simulink model "MCVT_v6_shell"  (R2021b)
settings: Solver=FixedStepAuto  StartTime=0.0  StopTime=1000000  FixedStep=1/fz  RelTol=1e-3
undefined symbols (not defined in the file or in its folder): fz_3
libraries: lib_subframe x71, slrealtimeutilitieslib x30, lib_header x15, slrealtimeiplib x15
(part 2 of 2)

== matlab function MCVT_v6_shell/Sys3_Power/Sys3_FDDs/3003003 ==
  settings: updateMethod=DISCRETE  sampleTime=1/fz_3
  data: fddmeas output
function fddmeas = FDD_model()

    fddmeas = rand(1,1);
    
end

== matlab function MCVT_v6_shell/Sys2_Structure/Sys2_Sensors/2002 ==
  settings: updateMethod=DISCRETE  sampleTime=1/fz_2
  data: meas output; fdd1 output; fdd2 output; fdd3 output
function [meas, fdd1, fdd2, fdd3] = Sensor_Model()
    
    meas = rand();
    fdd1 = randi([0 1]);
    fdd2 = rand();
    fdd3 = randi([0 1]);
    
end

== matlab function MCVT_v6_shell/Sys2_Structure/Sys2_Sensors/2005 ==
  settings: updateMethod=DISCRETE  sampleTime=1/fz_2
  data: meas output; fdd1 output; fdd2 output; fdd3 output
function [meas, fdd1, fdd2, fdd3] = Sensor_Model()
    
    meas = rand();
    fdd1 = randi([0 1]);
    fdd2 = rand();
    fdd3 = randi([0 1]);
    
end

== matlab function MCVT_v6_shell/Sys3_Power/Sys3_FDDs/3003004 ==
  settings: updateMethod=DISCRETE  sampleTime=1/fz_3
  data: fddmeas output
function fddmeas = FDD_model()

    fddmeas = rand(1,1);
    
end

== matlab function MCVT_v6_shell/Sys5_ECLSS/Sys5_FDDs/5002002 ==
  settings: updateMethod=DISCRETE  sampleTime=1/fz_5
  data: fddmeas output
function fddmeas = FDD_model()

    fddmeas = rand(1,1);
    
end

== matlab function MCVT_v6_shell/Sys3_Power/Sys3_Sensors/3004 ==
  settings: updateMethod=DISCRETE  sampleTime=1/fz_3
  data: meas output; fdd1 output; fdd2 output; fdd3 output
function [meas, fdd1, fdd2, fdd3] = Sensor_Model()
    
    meas = rand();
    fdd1 = randi([0 1]);
    fdd2 = rand();
    fdd3 = randi([0 1]);
    
end

== matlab function MCVT_v6_shell/Sys3_Power/Sys3_Sensors/3005 ==
  settings: updateMethod=DISCRETE  sampleTime=1/fz_3
  data: meas output; fdd1 output; fdd2 output; fdd3 output
function [meas, fdd1, fdd2, fdd3] = Sensor_Model()
    
    meas = rand();
    fdd1 = randi([0 1]);
    fdd2 = rand();
    fdd3 = randi([0 1]);
    
end

== matlab function MCVT_v6_shell/Sys3_Power/Sys3_Sensors/3006 ==
  settings: updateMethod=DISCRETE  sampleTime=1/fz_3
  data: meas output; fdd1 output; fdd2 output; fdd3 output
function [meas, fdd1, fdd2, fdd3] = Sensor_Model()
    
    meas = rand();
    fdd1 = randi([0 1]);
    fdd2 = rand();
    fdd3 = randi([0 1]);
    
end

== matlab function MCVT_v6_shell/Sys2_Structure/Sys2_Sensors/2006 ==
  settings: updateMethod=DISCRETE  sampleTime=1/fz_2
  data: meas output; fdd1 output; fdd2 output; fdd3 output
function [meas, fdd1, fdd2, fdd3] = Sensor_Model()
    
    meas = rand();
    fdd1 = randi([0 1]);
    fdd2 = rand();
    fdd3 = randi([0 1]);
    
end

== matlab function MCVT_v6_shell/Sys2_Structure/Sys2_Sensors/2003 ==
  settings: updateMethod=DISCRETE  sampleTime=1/fz_2
  data: meas output; fdd1 output; fdd2 output; fdd3 output
function [meas, fdd1, fdd2, fdd3] = Sensor_Model()
    
    meas = rand();
    fdd1 = randi([0 1]);
    fdd2 = rand();
    fdd3 = randi([0 1]);
    
end

== matlab function MCVT_v6_shell/Sys2_Structure/Sys2_Sensors/2004 ==
  settings: updateMethod=DISCRETE  sampleTime=1/fz_2
  data: meas output; fdd1 output; fdd2 output; fdd3 output
function [meas, fdd1, fdd2, fdd3] = Sensor_Model()
    
    meas = rand();
    fdd1 = randi([0 1]);
    fdd2 = rand();
    fdd3 = randi([0 1]);
    
end

== matlab function MCVT_v6_shell/Sys3_Power/Sys3_Sensors/3007 ==
  settings: updateMethod=DISCRETE  sampleTime=1/fz_3
  data: meas output; fdd1 output; fdd2 output; fdd3 output
function [meas, fdd1, fdd2, fdd3] = Sensor_Model()
    
    meas = rand();
    fdd1 = randi([0 1]);
    fdd2 = rand();
    fdd3 = randi([0 1]);
    
end

== matlab function MCVT_v6_shell/Sys5_ECLSS/Sys5_FDDs/5002003 ==
  settings: updateMethod=DISCRETE  sampleTime=1/fz_5
  data: fddmeas output
function fddmeas = FDD_model()

    fddmeas = rand(1,1);
    
end

== matlab function MCVT_v6_shell/Sys3_Power/Sys3_Sensors/3011 ==
  settings: updateMethod=DISCRETE  sampleTime=1/fz_3
  data: meas output; fdd1 output; fdd2 output; fdd3 output
function [meas, fdd1, fdd2, fdd3] = Sensor_Model()
    
    meas = rand();
    fdd1 = randi([0 1]);
    fdd2 = rand();
    fdd3 = randi([0 1]);
    
end

== matlab function MCVT_v6_shell/Sys3_Power/Sys3_Sensors/3010 ==
  settings: updateMethod=DISCRETE  sampleTime=1/fz_3
  data: meas output; fdd1 output; fdd2 output; fdd3 output
function [meas, fdd1, fdd2, fdd3] = Sensor_Model()
    
    meas = rand();
    fdd1 = randi([0 1]);
    fdd2 = rand();
    fdd3 = randi([0 1]);
    
end

== matlab function MCVT_v6_shell/Sys3_Power/Sys3_Sensors/3009 ==
  settings: updateMethod=DISCRETE  sampleTime=1/fz_3
  data: meas output; fdd1 output; fdd2 output; fdd3 output
function [meas, fdd1, fdd2, fdd3] = Sensor_Model()
    
    meas = rand();
    fdd1 = randi([0 1]);
    fdd2 = rand();
    fdd3 = randi([0 1]);
    
end

== matlab function MCVT_v6_shell/Sys3_Power/Sys3_Sensors/3008 ==
  settings: updateMethod=DISCRETE  sampleTime=1/fz_3
  data: meas output; fdd1 output; fdd2 output; fdd3 output
function [meas, fdd1, fdd2, fdd3] = Sensor_Model()
    
    meas = rand();
    fdd1 = randi([0 1]);
    fdd2 = rand();
    fdd3 = randi([0 1]);
    
end

== matlab function MCVT_v6_shell/Sys3_Power/Sys3_Sensors/3012 ==
  settings: updateMethod=DISCRETE  sampleTime=1/fz_3
  data: meas output; fdd1 output; fdd2 output; fdd3 output
function [meas, fdd1, fdd2, fdd3] = Sensor_Model()
    
    meas = rand();
    fdd1 = randi([0 1]);
    fdd2 = rand();
    fdd3 = randi([0 1]);
    
end

== matlab function MCVT_v6_shell/Sys3_Power/Sys3_Sensors/3013 ==
  settings: updateMethod=DISCRETE  sampleTime=1/fz_3
  data: meas output; fdd1 output; fdd2 output; fdd3 output
function [meas, fdd1, fdd2, fdd3] = Sensor_Model()
    
    meas = rand();
    fdd1 = randi([0 1]);
    fdd2 = rand();
    fdd3 = randi([0 1]);
    
end

== matlab function MCVT_v6_shell/Sys5_ECLSS/Sys5_FDDs/5002004 ==
  settings: updateMethod=DISCRETE  sampleTime=1/fz_5
  data: fddmeas output
function fddmeas = FDD_model()

    fddmeas = rand(1,1);
    
end

== matlab function MCVT_v6_shell/Sys3_Power/Sys3_Sensors/3014 ==
  settings: updateMethod=DISCRETE  sampleTime=1/fz_3
  data: meas output; fdd1 output; fdd2 output; fdd3 output
function [meas, fdd1, fdd2, fdd3] = Sensor_Model()
    
    meas = rand();
    fdd1 = randi([0 1]);
    fdd2 = rand();
    fdd3 = randi([0 1]);
    
end

== matlab function MCVT_v6_shell/Sys3_Power/Sys3_FDDs/3003005 ==
  settings: updateMethod=DISCRETE  sampleTime=1/fz_3
  data: fddmeas output
function fddmeas = FDD_model()

    fddmeas = rand(1,1);
    
end

== matlab function MCVT_v6_shell/Sys3_Power/Sys3_FDDs/3003006 ==
  settings: updateMethod=DISCRETE  sampleTime=1/fz_3
  data: fddmeas output
function fddmeas = FDD_model()

    fddmeas = rand(1,1);
    
end

== matlab function MCVT_v6_shell/Sys3_Power/Sys3_FDDs/3003007 ==
  settings: updateMethod=DISCRETE  sampleTime=1/fz_3
  data: fddmeas output
function fddmeas = FDD_model()

    fddmeas = rand(1,1);
    
end

== matlab function MCVT_v6_shell/Sys5_ECLSS/Sys5_FDDs/5003001 ==
  settings: updateMethod=DISCRETE  sampleTime=1/fz_5
  data: fddmeas output
function fddmeas = FDD_model()

    fddmeas = rand(1,1);
    
end

== matlab function MCVT_v6_shell/Sys5_ECLSS/Sys5_FDDs/5003002 ==
  settings: updateMethod=DISCRETE  sampleTime=1/fz_5
  data: fddmeas output
function fddmeas = FDD_model()

    fddmeas = rand(1,1);
    
end

== matlab function MCVT_v6_shell/Sys5_ECLSS/Sys5_FDDs/5003003 ==
  settings: updateMethod=DISCRETE  sampleTime=1/fz_5
  data: fddmeas output
function fddmeas = FDD_model()

    fddmeas = rand(1,1);
    
end

== matlab function MCVT_v6_shell/Sys5_ECLSS/Sys5_FDDs/5003004 ==
  settings: updateMethod=DISCRETE  sampleTime=1/fz_5
  data: fddmeas output
function fddmeas = FDD_model()

    fddmeas = rand(1,1);
    
end

== matlab function MCVT_v6_shell/Sys5_ECLSS/Sys5_Sensors/5005 ==
  settings: updateMethod=DISCRETE  sampleTime=1/fz_5
  data: meas output; fdd1 output; fdd2 output; fdd3 output
function [meas, fdd1, fdd2, fdd3] = Sensor_Model()
    
    meas = rand();
    fdd1 = randi([0 1]);
    fdd2 = rand();
    fdd3 = randi([0 1]);
    
end

== matlab function MCVT_v6_shell/Sys5_ECLSS/Sys5_Sensors/5006 ==
  settings: updateMethod=DISCRETE  sampleTime=1/fz_5
  data: meas output; fdd1 output; fdd2 output; fdd3 output
function [meas, fdd1, fdd2, fdd3] = Sensor_Model()
    
    meas = rand();
    fdd1 = randi([0 1]);
    fdd2 = rand();
    fdd3 = randi([0 1]);
    
end

== matlab function MCVT_v6_shell/Sys5_ECLSS/Sys5_Sensors/5007 ==
  settings: updateMethod=DISCRETE  sampleTime=1/fz_5
  data: meas output; fdd1 output; fdd2 output; fdd3 output
function [meas, fdd1, fdd2, fdd3] = Sensor_Model()
    
    meas = rand();
    fdd1 = randi([0 1]);
    fdd2 = rand();
    fdd3 = randi([0 1]);
    
end

== matlab function MCVT_v6_shell/Sys5_ECLSS/Sys5_Sensors/5008 ==
  settings: updateMethod=DISCRETE  sampleTime=1/fz_5
  data: meas output; fdd1 output; fdd2 output; fdd3 output
function [meas, fdd1, fdd2, fdd3] = Sensor_Model()
    
    meas = rand();
    fdd1 = randi([0 1]);
    fdd2 = rand();
    fdd3 = randi([0 1]);
    
end
